simulink library "waijung_addon_module"  (R2015b)
settings: Solver=ode45  StartTime=0.0  StopTime=10.0  RelTol=1e-3
libraries: simulink x2
settings Model: Creator=Krisada  LastModifiedBy=Aimagin
settings DataIOCC: SaveFormat=Array  SignalLoggingSaveFormat=ModelDataLogs
settings OptimizationCC: ExpressionDepthLimit=2147483647
settings DebuggingCC: UnderspecifiedInitializationDetection=Classic  MergeDetectMultiDrivingBlocksExec=none  SolverPrmCheckMsg=warning  FcnCallInpInsideContextMsg=UseLocalSettings  StateNameClashWarn=warning  StrictBusMsg=Warning
settings HardwareCC: ProdBitPerPointer=32  ProdLargestAtomicFloat=None  ProdIntDivRoundTo=Undefined  ProdEndianess=Unspecified  ProdWordSize=32  ProdHWDeviceType=32-bit Generic
settings GRTTargetCC: CombineOutputUpdateFcns=off  GRTInterface=on
settings ConfigComp: CovModelRefEnable=Off

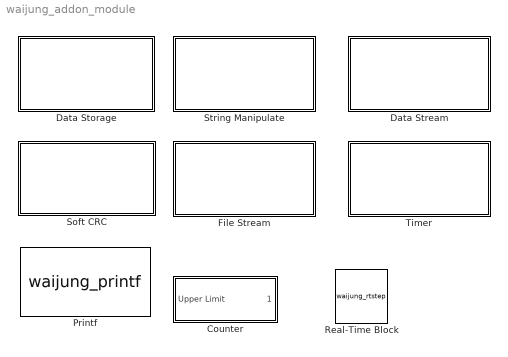
== system waijung_addon_module ==
  Counter : Subsystem  mask(waijung_counter){}
      mask help: This block outputs counter from zero to upper limit. The output is incremented by one every sample time. The sample time can be inherited from input upper limit sampletime.
  Data Storage : Subsystem
      mask Display: disp('Data Storage');
  Data Stream : Subsystem
      settings: OpenFcn=waijung_data_stream_lib
      mask Display: disp('Data Stream');
  File Stream : Subsystem
      settings: OpenFcn=waijung_filestream_lib
      mask Display: disp('File Stream');
  Printf : S-Function  FunctionName=waijung_printf  Parameters=storagename,printfformat,formatcode,varname,sampletime,sampletimestr,blockid  SFunctionDeploymentMode=off  EnableBusSupport=off  mask(waijung_printf){storagename=D0, printfformat=%d,%u, formatcode=du, varname=, sampletime=-1, sampletimestr=0, blockid=Printf}
      mask prompts: storagename "Storage Name"; printfformat "Printf format"; formatcode "Printf format code"; varname "Variable name"; sampletime "Sample time (sec)"; sampletimestr "Compiled sample time (sec) in string"
      mask help: This block implements printf command.
      mask init:
      | waijung_printf_callback('init');
      mask Help: web(fullfile(waijungdocroot,'waijung_printf.htm'))
      mask TypeOptions storagename: S | D0
      mask Callback storagename: waijung_printf_callback('storagename');
      mask Callback printfformat: waijung_printf_callback('printfformat');
      mask Callback formatcode: waijung_printf_callback('formatcode');
      mask Callback varname: waijung_printf_callback('varname');
      mask Callback sampletime: waijung_printf_callback('sampletime');
      mask Callback sampletimestr: waijung_printf_callback('sampletimestr');
      mask Callback blockid: waijung_printf_callback('blockid');
      mask Display: text(0.95, 0.5, 'Buffer: D0\nTs (sec): 0','ver','middle','hor','right');port_label('input',1,'D1(%d)');port_label('input',2,'D2(%u)');
  Real-Time Block : M-S-Function  Priority=0  FunctionName=waijung_rtstep  mask(waijung_rtstep){setting=Default, sampletime=-1}
      mask prompts: sampletime "Sample time (sec)"
      mask help:
      | Make Simulink simulation step in near real-time.
      |
      | Default: Sample time is determined automatically using system base sample time (smallest sample time).
      |
      | Custom: Manually input sample time.
      mask init:
      | waijung_rtstep_callback('init');
      mask TypeOptions setting: Default | Custom
      mask Callback setting: waijung_rtstep_callback('setting');
      mask Callback sampletime: waijung_rtstep_callback;
      mask Display: text(0.5,0.5,'RT Step\n-1\nsec','hor','center','ver','middle')
  Soft CRC : Subsystem
      settings: OpenFcn=waijung_crc_lib
      mask Display: disp('Soft CRC');
  String Manipulate : Subsystem
      settings: OpenFcn=waijung_string_manipulate
      mask Display: disp('String Manipulate');
  Timer : Subsystem
      settings: OpenFcn=waijung_systimer_lib
      mask Display: disp('Timer');

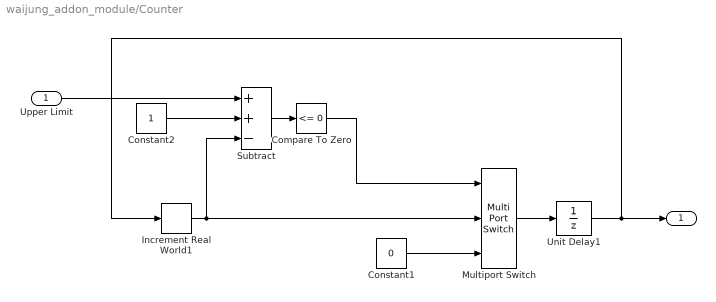
== system waijung_addon_module/Counter ==
  Upper Limit : Inport
  Compare To Zero : simulink/Logic and Bit Operations/Compare To Zero  SystemSampleTime=-1  relop=<=  LogicOutDataTypeMode=uint8
  Constant1 : Constant  Value=0
  Constant2 : Constant
  Increment Real World1 : simulink/Additional Math & Discrete/Additional Math: Increment - Decrement/Increment Real World  SystemSampleTime=-1
  Multiport Switch : MultiPortSwitch  DataPortOrder=Zero-based contiguous  Inputs=2  zeroidx=on
  Subtract : Sum  Inputs=++-
  Unit Delay1 : UnitDelay  SampleTime=-1
  " " : Outport
  wires:
  Unit Delay1/1 -> Increment Real World1/1, " "/1
  Multiport Switch/1 -> Unit Delay1/1
  Increment Real World1/1 -> Multiport Switch/2, Subtract/3
  Subtract/1 -> Compare To Zero/1
  Constant1/1 -> Multiport Switch/3
  Compare To Zero/1 -> Multiport Switch/1
  Upper Limit/1 -> Subtract/1
  Constant2/1 -> Subtract/2

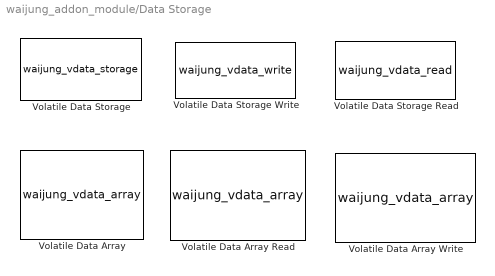
== system waijung_addon_module/Data Storage ==
  Volatile Data Array : S-Function  FunctionName=waijung_vdata_array  Parameters=conf,inputporttype,inputportwidth,outputporttype,outputportwidth,optionstring,sampletime,blockid  SFunctionDeploymentMode=off  EnableBusSupport=off  mask(waijung_vdata_array){conf=Setup, specificaddress=off, storagename=Array1, memoryaddress=hex2dec('64000000'), storagetype=uint8, datasize=120*160, varname=VolatileDataArray_Array1, datatype=double, datacount=0, portpinstr=0, sampletime=-1, blockid=DataStorageVolatileDataArray, inputporttype=[], inputportwidth=[], inputportlabel={}, outputporttype=[], outputportwidth=[], outputportlabel={}, compat=0, optionstring=[]}
      mask prompts: conf "Configuration"; specificaddress "Specific Memory Address"; storagename "Array Name"; memoryaddress "Memory address"; storagetype "Array Data Type"; datasize "Array Size"; varname "Variable name"; datatype "Data type"; datacount "Data count"; portpinstr "Port Pin String"; sampletime "Sample time (sec)"; blockid "Block ID"; inputporttype "Input Port Type"; inputportwidth "Input Port Width"; inputportlabel "Input Port Label"; outputporttype "Output Port Type"; outputportwidth "Output Port Width"; outputportlabel "Output port label"; compat "Compatibility (Reserved for future use)"; optionstring "String(s) to be passed to TLC"
      mask init:
      | waijung_vdata_array_callback('init');
      mask Help: web(fullfile(waijungdocroot,'waijung_vdata_array.htm'), '-browser')
      mask TypeOptions conf: Setup | Read
      mask Callback conf: waijung_vdata_array_callback('conf');
      mask Callback specificaddress: waijung_vdata_array_callback('specificaddress');
      mask Callback storagename: waijung_vdata_array_callback('storagename');
      mask TypeOptions storagetype: double | single | uint32 | int32 | uint16 | int16 | uint8 | int8
      mask TypeOptions datatype: double | single | int8 | uint8 | int16 | uint16 | int32 | uint32
      mask Callback sampletime: waijung_vdata_array_callback('sampletime');
      mask Callback blockid: waijung_vdata_array_callback('blockid');
      mask Display: text(0.5, 0.5, '[Array Setup]\nName: Array1\nSize: 19200','ver','middle','hor','center');
  Volatile Data Array Read : S-Function  FunctionName=waijung_vdata_array  Parameters=conf,inputporttype,inputportwidth,outputporttype,outputportwidth,optionstring,sampletime,blockid  SFunctionDeploymentMode=off  EnableBusSupport=off  mask(waijung_vdata_array){conf=Read, specificaddress=off, storagename=Array1, memoryaddress=hex2dec('64000000'), storagetype=uint8, datasize=120*160*3, varname=VolatileDataArray_Array1, datatype=uint8, datacount=128, variablesize=off, portpinstr=0, sampletime=-1, blockid=DataStorageVolatileDataArrayRead, inputporttype=[7], inputportwidth=[1], inputportlabel={'Offset'}, outputporttype=[3], outputportwidth=[128], outputportlabel={'Data(128)'}, compat=0, optionstring=[]}
      mask prompts: conf "Configuration"; specificaddress "Specific Memory Address"; storagename "Array Name"; memoryaddress "Memory address"; storagetype "Array Data Type"; datasize "Array Size (bytes)"; varname "Variable name"; datatype "Data type"; datacount "Data count"; variablesize "Variable size"; portpinstr "Port Pin String"; sampletime "Sample time (sec)"; blockid "Block ID"; inputporttype "Input Port Type"; inputportwidth "Input Port Width"; inputportlabel "Input Port Label"; outputporttype "Output Port Type"; outputportwidth "Output Port Width"; outputportlabel "Output port label"; compat "Compatibility (Reserved for future use)"; optionstring "String(s) to be passed to TLC"
      mask init:
      | waijung_vdata_array_callback('init');
      mask Help: web(fullfile(waijungdocroot,'waijung_vdata_array.htm'), '-browser')
      mask TypeOptions conf: Setup | Read | Write
      mask Callback conf: waijung_vdata_array_callback('conf');
      mask Callback specificaddress: waijung_vdata_array_callback('specificaddress');
      mask Callback storagename: waijung_vdata_array_callback('storagename');
      mask TypeOptions storagetype: double | single | uint32 | int32 | uint16 | int16 | uint8 | int8
      mask TypeOptions datatype: double | single | int8 | uint8 | int16 | uint16 | int32 | uint32
      mask Callback variablesize: waijung_vdata_array_callback('variablesize');
      mask Callback sampletime: waijung_vdata_array_callback('sampletime');
      mask Callback blockid: waijung_vdata_array_callback('blockid');
      mask Display: text(0.5, 0.5, '[Array Read]\nName: Array1\nType: uint8\nSize: 128\nTs (sec): 0','ver','middle','hor','center'); port_label('input', 1,'Offset'); port_label('output', 1,'Data(128)');
  Volatile Data Array Write : S-Function  FunctionName=waijung_vdata_array  Parameters=conf,inputporttype,inputportwidth,outputporttype,outputportwidth,optionstring,sampletime,blockid  SFunctionDeploymentMode=off  EnableBusSupport=off  mask(waijung_vdata_array){conf=Write, specificaddress=off, storagename=Array1, memoryaddress=hex2dec('64000000'), storagetype=uint8, datasize=120*160*3, varname=VolatileDataArray_Array1, datatype=uint8, datacount=128, variablesize=off, portpinstr=0, sampletime=-1, blockid=DataStorageVolatileDataArrayWrite, inputporttype=[7 3], inputportwidth=[1 128], inputportlabel={'Offset', 'Data'}, outputporttype=[], outputportwidth=[], outputportlabel={}, compat=0, optionstring=[]}
      mask prompts: conf "Configuration"; specificaddress "Specific Memory Address"; storagename "Array Name"; memoryaddress "Memory address"; storagetype "Array Data Type"; datasize "Array Size (bytes)"; varname "Variable name"; datatype "Data type"; datacount "Data count"; variablesize "Variable size"; portpinstr "Port Pin String"; sampletime "Sample time (sec)"; blockid "Block ID"; inputporttype "Input Port Type"; inputportwidth "Input Port Width"; inputportlabel "Input Port Label"; outputporttype "Output Port Type"; outputportwidth "Output Port Width"; outputportlabel "Output port label"; compat "Compatibility (Reserved for future use)"; optionstring "String(s) to be passed to TLC"
      mask init:
      | waijung_vdata_array_callback('init');
      mask Help: web(fullfile(waijungdocroot,'waijung_vdata_array.htm'), '-browser')
      mask TypeOptions conf: Setup | Read | Write
      mask Callback conf: waijung_vdata_array_callback('conf');
      mask Callback specificaddress: waijung_vdata_array_callback('specificaddress');
      mask Callback storagename: waijung_vdata_array_callback('storagename');
      mask TypeOptions storagetype: double | single | uint32 | int32 | uint16 | int16 | uint8 | int8
      mask TypeOptions datatype: double | single | int8 | uint8 | int16 | uint16 | int32 | uint32
      mask Callback variablesize: waijung_vdata_array_callback('variablesize');
      mask Callback sampletime: waijung_vdata_array_callback('sampletime');
      mask Callback blockid: waijung_vdata_array_callback('blockid');
      mask Display: text(0.95, 0.5, '[Array Write]\nName: Array1\nType: uint8\nSize: 128\nTs (sec): 0','ver','middle','hor','right'); port_label('input', 1,'Offset'); port_label('input', 2,'Data');
  Volatile Data Storage : S-Function  FunctionName=waijung_vdata_storage  Parameters=storagetype,storagename,initval,varname,buffersize,initvalstring,sampletime,sampletimestr,blockid,storagetypestr  SFunctionDeploymentMode=off  EnableBusSupport=off  mask(waijung_vdata_storage){storagetype=string, definevolatile=off, storagename=S, initval=0, varname=DataStorageVolatileDataStorage_S, buffersize=64, initvalstring='Initial string', webintegration=Disable, weboutputformat='%s', webcgicallback=(void*)0, laststoragetype=string, sampletime=-1, sampletimestr=0, blockid=DataStorageVolatileDataStorage, storagetypestr=char}
      mask prompts: storagetype "Storage Type"; definevolatile "Define with "volatile" keyword"; storagename "Storage Name (must be a valid variable name)"; initval "Initial value (Apply at Power on Reset only)"; varname "Variable name"; buffersize "Size (bytes)"; initvalstring "Initial value (Apply at Power on Reset only)"; webintegration "Web CGI varget/varset integration"; weboutputformat "Web CGI varget output format"; webcgicallback "Web CGI varset callback"; laststoragetype "Last selected Storage Type"; sampletime "Sample time (sec)"; sampletimestr "Compiled sample time (sec) in string"; storagetypestr "Type string"
      mask help:
      | This block implements a volatile Data Storage.
      |
      | Web CGI varset/varget integratiopn:
      | Enable - In webserver application, allow remote access via http.
      | Disable - Variable is use in local only.
      mask init:
      | waijung_vdata_storage_callback('init');
      mask Help: web(fullfile(waijungdocroot,'Volatile_Data_Storage.htm'))
      mask TypeOptions storagetype: double | single | uint32 | int32 | uint16 | int16 | uint8 | int8 | string
      mask Callback storagetype: waijung_vdata_storage_callback('storagetype');
      mask Callback storagename: waijung_vdata_storage_callback('storagename');
      mask Callback initval: waijung_vdata_storage_callback('initval');
      mask Callback varname: waijung_vdata_storage_callback('varname');
      mask Callback initvalstring: waijung_vdata_storage_callback('initvalstring');
      mask TypeOptions webintegration: Disable | ReadOnly | Write/ Read | ReadOnly with KeyValuePair | Write/ Read with KeyValuePair
      mask Callback webintegration: waijung_vdata_storage_callback('webintegration');
      mask Callback weboutputformat: waijung_vdata_storage_callback('weboutputformat');
      mask TypeOptions laststoragetype: double | single | uint32 | int32 | uint16 | int16 | uint8 | int8 | string
      mask Callback sampletime: waijung_vdata_storage_callback('sampletime');
      mask Callback sampletimestr: waijung_vdata_storage_callback('sampletimestr');
      mask Callback blockid: waijung_vdata_storage_callback('blockid');
      mask Display: text(0.5, 0.5, 'Name: S\nType: string','ver','middle','hor','center')
  Volatile Data Storage Read : S-Function  FunctionName=waijung_vdata_read  Parameters=storagename,varname,sampletime,sampletimestr,blockid,storagetype,storagetypestr  SFunctionDeploymentMode=off  EnableBusSupport=off  mask(waijung_vdata_read){storagename=S, varname=DataStorageVolatileDataStorage_S, sampletime=-1, sampletimestr=0, blockid=DataStorageVolatileDataStorageRead, storagetype=string, storagetypestr=uint32_t}
      mask prompts: storagename "Storage Name"; varname "Variable name"; sampletime "Sample time (sec)"; sampletimestr "Compiled sample time (sec) in string"; storagetype "Data type"; storagetypestr "Data type string"
      mask help: This block implements read data from a buffer.
      mask init:
      | waijung_vdata_read_callback('init');
      mask Help: web(fullfile(waijungdocroot,'Volatile_Data_Storage_Read.htm'))
      mask TypeOptions storagename: S
      mask Callback storagename: waijung_vdata_read_callback('storagename');
      mask Callback varname: waijung_vdata_read_callback('varname');
      mask Callback sampletime: waijung_vdata_read_callback('sampletime');
      mask Callback sampletimestr: waijung_vdata_read_callback('sampletimestr');
      mask Callback blockid: waijung_vdata_read_callback('blockid');
      mask Callback storagetype: waijung_vdata_read_callback('storagetype');
      mask Display: text(0.05, 0.5, 'Buffer: S','ver','middle','hor','left');port_label('output',1,'D1(string)')
  Volatile Data Storage Write : S-Function  FunctionName=waijung_vdata_write  Parameters=storagename,varname,sampletime,sampletimestr,blockid,storagetype,storagetypestr  SFunctionDeploymentMode=off  EnableBusSupport=off  mask(waijung_vdata_write){storagename=S, varname=DataStorageVolatileDataStorage_S, sampletime=-1, sampletimestr=0, blockid=DataStorageVolatileDataStorageWrite, storagetype=string, storagetypestr=char*}
      mask prompts: storagename "Storage Name"; varname "Variable name"; sampletime "Sample time (sec)"; sampletimestr "Compiled sample time (sec) in string"; storagetype "Data type"; storagetypestr "Data type string"
      mask help: This block implements write data to a buffer.
      mask init:
      | waijung_vdata_write_callback('init');
      mask Help: web(fullfile(waijungdocroot,'Volatile_Data_Storage_Write.htm'))
      mask TypeOptions storagename: S
      mask Callback storagename: waijung_vdata_write_callback('storagename');
      mask Callback varname: waijung_vdata_write_callback('varname');
      mask Callback sampletime: waijung_vdata_write_callback('sampletime');
      mask Callback sampletimestr: waijung_vdata_write_callback('sampletimestr');
      mask Callback blockid: waijung_vdata_write_callback('blockid');
      mask Callback storagetype: waijung_vdata_write_callback('storagetype');
      mask Display: text(0.95, 0.5, 'Buffer: S','ver','middle','hor','right');port_label('input',1,'D1(string)')

== system waijung_addon_module/Data Stream ==

== system waijung_addon_module/File Stream ==

== system waijung_addon_module/Soft CRC ==

== system waijung_addon_module/String Manipulate ==

== system waijung_addon_module/Timer ==
